simulink model "fir8_03"  (R2019b)
settings: Solver=FixedStepDiscrete  StartTime=0.0  StopTime=3000  RelTol=1e-3
settings Model: Creator=moeller  LastModifiedBy=bhisma
settings DataIOCC: LimitDataPoints=on  SaveFormat=Array  SignalLoggingSaveFormat=ModelDataLogs  ReturnWorkspaceOutputs=off
settings OptimizationCC: BlockReduction=off  ConditionallyExecuteInputs=off  ExpressionDepthLimit=2147483647  LifeSpan=inf
settings DebuggingCC: UnderspecifiedInitializationDetection=Classic  MergeDetectMultiDrivingBlocksExec=none  SolverPrmCheckMsg=warning  MultiTaskCondExecSysMsg=warning  SingleTaskRateTransMsg=error  FcnCallInpInsideContextMsg=warning  StateNameClashWarn=warning  SFUnexpectedBacktrackingDiag=warning  SFNoUnconditionalDefaultTransitionDiag=warning  SFExecutionAtInitializationDiag=none  ArithmeticOperatorsInVariantConditions=warning
settings HardwareCC: ProdBitPerPointer=32  ProdBitPerSizeT=32  ProdBitPerPtrDiffT=32  ProdLargestAtomicFloat=None  ProdIntDivRoundTo=Undefined  ProdEndianess=Unspecified  ProdWordSize=32  ProdHWDeviceType=32-bit Generic
settings ModelReferenceCC: PropagateSignalLabelsOutOfModel=off
settings SFSimCC: SimUseLocalCustomCode=off  CustomCodeUndefinedFunction=UseInterfaceOnly
settings RTWCC: RTWUseLocalCustomCode=off
settings CodeAppCC: StateflowObjectComments=on
settings GRTTargetCC: TargetLangStandard=C89/C90 (ANSI)  GeneratePreprocessorConditionals=Disable all  CombineOutputUpdateFcns=off  GRTInterface=on
settings ConfigComp: CovMetricSettings=dw  CovHtmlReporting=on  CovSaveCumulativeToWorkspaceVar=on  CovSaveSingleToWorkspaceVar=on  CovExternalEMLEnable=off  CovSFcnEnable=off

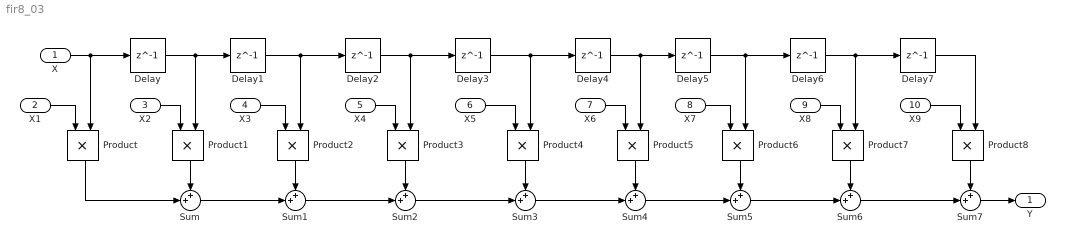
== system fir8_03 ==
  X : Inport
  X1 : Inport  Port=2  OutDataTypeStr=fixdt(1,32,16)
  X2 : Inport  Port=3  OutDataTypeStr=fixdt(1,32,16)
  X3 : Inport  Port=4  OutDataTypeStr=fixdt(1,32,16)
  X4 : Inport  Port=5  OutDataTypeStr=fixdt(1,32,16)
  X5 : Inport  Port=6  OutDataTypeStr=fixdt(1,32,16)
  X6 : Inport  Port=7  OutDataTypeStr=fixdt(1,32,16)
  X7 : Inport  Port=8  OutDataTypeStr=fixdt(1,32,16)
  X8 : Inport  Port=9  OutDataTypeStr=fixdt(1,32,16)
  X9 : Inport  Port=10  OutDataTypeStr=fixdt(1,32,16)
  Delay{,1..7} (8 alike) : Delay  DelayLength=1  SampleTime=1
  Product{,1..8} (9 alike) : Product  OutDataTypeStr=fixdt(1,32,16)  RndMeth=Zero
  Sum{,1..7} (8 alike) : Sum  Inputs=++|  AccumDataTypeStr=fixdt(1,32,16)  OutDataTypeStr=fixdt(1,32,16)
  Y : Outport  OutDataTypeStr=fixdt(1,32,16)
  wires:
  X/1 -> Delay/1, Product/2
  X1/1 -> Product/1
  Product/1 -> Sum/2
  X2/1 -> Product1/1
  Product1/1 -> Sum/1
  Delay/1 -> Delay1/1, Product1/2
  X3/1 -> Product2/1
  Delay1/1 -> Delay2/1, Product2/2
  X4/1 -> Product3/1
  Delay2/1 -> Product3/2, Delay3/1
  Product2/1 -> Sum1/1
  Sum/1 -> Sum1/2
  Sum1/1 -> Sum2/2
  Product3/1 -> Sum2/1
  Sum2/1 -> Sum3/2
  Product4/1 -> Sum3/1
  X5/1 -> Product4/1
  Delay3/1 -> Product4/2, Delay4/1
  X6/1 -> Product5/1
  Product5/1 -> Sum4/1
  Delay4/1 -> Delay5/1, Product5/2
  X7/1 -> Product6/1
  Delay5/1 -> Delay6/1, Product6/2
  X8/1 -> Product7/1
  Delay6/1 -> Product7/2, Delay7/1
  Product6/1 -> Sum5/1
  Sum4/1 -> Sum5/2
  Sum5/1 -> Sum6/2
  Product7/1 -> Sum6/1
  Sum6/1 -> Sum7/2
  Product8/1 -> Sum7/1
  X9/1 -> Product8/1
  Delay7/1 -> Product8/2
  Sum3/1 -> Sum4/2
  Sum7/1 -> Y/1
